simulink model "fxpdemo_prelookup_utilfcn"  (Simulink 7.6)
settings: Solver=FixedStepDiscrete  StartTime=0.0  StopTime=0.01  FixedStep=0.01  RelTol=1e-3
PreLoadFcn:
  | tabledata=Simulink.Parameter;
  | tabledata.RTWInfo.StorageClass = 'ExportedGlobal';
  | tabledata.DataType='fixdt(0,8,6)';
  | tabledata.Value=sin(linspace(0,pi,10));
Description:
  | Shared Utility Functions for Prelookup Blocks
  | The utility functions generated by the Prelookup block are determined by the target
  | data type of the block's inputs, outputs, and breakpoint parameter, as well as the
  | *Index search method* and *Integer rounding mode*. Even if the two Prelookup blocks
  | in this model have different data types, they fullfill the above requirements and
  | share their utility functions.
  | 
  | To see this in the generated code, open the model and build it.
settings Model: Creator=The MathWorks Inc.
settings DataIOCC: SaveFormat=StructureWithTime
settings OptimizationCC: InlineParams=on  OptimizeModelRefInitCode=on  LifeSpan=1
settings DebuggingCC: ParameterPrecisionLossMsg=none  StrictBusMsg=Warning
settings HardwareCC: ProdBitPerLong=64  ProdHWDeviceType=Generic->Custom
settings RTWCC: SystemTargetFile=ert.tlc  GenCodeOnly=on  TemplateMakefile=ert_default_tmf  Description=Real-Time Workshop Embedded Coder (no auto configuration)  GenerateReport=on  RTWVerbose=off  ProcessScript=ert_make_rtw_hook  IncludeHyperlinkInReport=on  LaunchReport=on
settings CodeAppCC: IgnoreCustomStorageClasses=off
settings ERTTargetCC: MultiwordLength=2048  GenerateSampleERTMain=on  ERTCustomFileTemplate=example_file_process.tlc  ConvertIfToSwitch=off

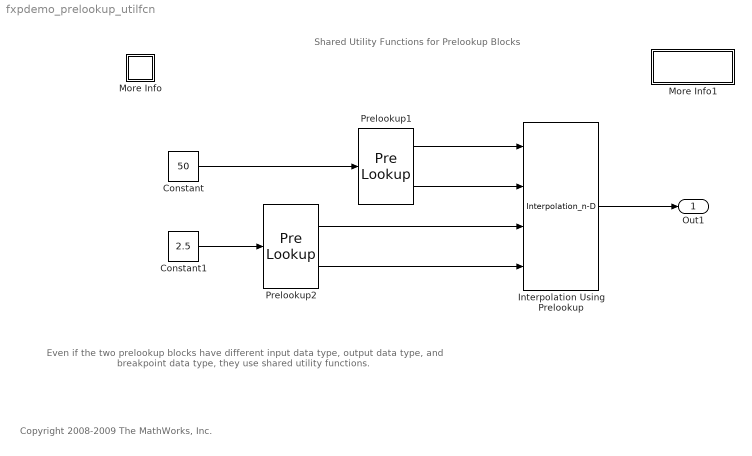
== system fxpdemo_prelookup_utilfcn ==
  note: Copyright 2008-2009 The MathWorks, Inc.
  note: Even if the two prelookup blocks have different input data type, output data
      | type, and breakpoint data type, they use shared utility functions.
  note: Shared Utility Functions for Prelookup Blocks
  Constant : Constant  Value=50  OutDataTypeStr=fixdt(0,32,8)  SampleTime=0.01
  Constant1 : Constant  Value=2.5  OutDataTypeStr=fixdt(0,20,8)  SampleTime=0.01
  Interpolation Using Prelookup : Interpolation_n-D  Table=[1:11]'*[1:11]  ExtrapMethod=None - Clip  OutDataTypeStr=fixdt(1,32,16)  TableDataTypeStr=fixdt(1,16,4)
  More Info : Subsystem
      settings: OpenFcn=showdemo(bdroot(gcs))
      mask Display: disp('?')
  More Info1 : Subsystem
      settings: OpenFcn=rtwbuild(bdroot(gcs))
      mask Display: fprintf('Double-click to\ngenerate code')
  Prelookup1 : PreLookup  BreakpointsData=[10:10:110]  BreakpointDataTypeStr=fixdt(1,26,0)  IndexDataTypeStr=fixdt(1,15)  FractionDataTypeStr=fixdt(1,27,12)
      settings: AttributesFormatString=Breakpoint data type = %<BreakpointDataTypeStr>
  Prelookup2 : PreLookup  BreakpointsData=[0:1:10]  BreakpointDataTypeStr=fixdt(1,20,0)  IndexDataTypeStr=fixdt(1,14)  FractionDataTypeStr=fixdt(1,30,12)
      settings: AttributesFormatString=Breakpoint data type = %<BreakpointDataTypeStr>
  Out1 : Outport
  wires:
  Constant/1 -> Prelookup1/1
  Prelookup1/1 -> Interpolation Using Prelookup/1
  Prelookup1/2 -> Interpolation Using Prelookup/2
  Interpolation Using Prelookup/1 -> Out1/1
  Constant1/1 -> Prelookup2/1
  Prelookup2/1 -> Interpolation Using Prelookup/3
  Prelookup2/2 -> Interpolation Using Prelookup/4

== system fxpdemo_prelookup_utilfcn/More Info ==

== system fxpdemo_prelookup_utilfcn/More Info1 ==
